simulink model "L400_airframe"  (R2024b)
settings: Solver=FixedStepAuto  StartTime=0  StopTime=20  FixedStep=5/1000  RelTol=1e-3
model workspace (MAT data in the model file):
  Sig : Simulink.Signal (value not decoded)
  Sig1 : Simulink.Signal (value not decoded)
  Sig2 : Simulink.Signal (value not decoded)
  Sig3 : Simulink.Signal (value not decoded)
  Sig4 : Simulink.Signal (value not decoded)
  Sig5 : Simulink.Signal (value not decoded)
  Sig6 : Simulink.Signal (value not decoded)
undefined symbols (not defined in the file or in its folder): convertTo, datetime, db, Earth, F, lambda, Light, MIL, WGS84, WMM2020
libraries: aerolibconvert2 x16, aerolibasang x5, aerolibtransform2 x3, aerolibwind2 x3, aerolibactuator x2, matrix_library x2, shared6dof x1, aerolibatmos2 x1, aerolibgravity2 x1
(part 2 of 4)

== system L400_airframe/actuator/aerodynamic/actuator ==
  BusElementIn1 : Inport  PortName=command  Element=DAL
  BusElementIn : Inport  PortName=command  Element=DAL
  BusElementIn2 : Inport  PortName=command  Element=DER
  BusElementIn3 : Inport  PortName=command  Element=DR
  BusElementIn4 : Inport  PortName=command  Element=DEM
  BusElementIn5 : Inport  PortName=command  Element=DEL
  BusElementIn6 : Inport  PortName=command  Element=DFLO
  BusElementIn7 : Inport  PortName=command  Element=DFLI
  BusElementIn8 : Inport  PortName=command  Element=DFRI
  BusElementIn9 : Inport  PortName=command  Element=DFRO
  Data Type Conversion : DataTypeConversion  SaturateOnIntegerOverflow=off  RndMeth=Floor
  Demux : Demux  Outputs=10
  Mux : Mux  Inputs=10
  Saturation : Saturate  UpperLimit=[30,30,30,30,15,15,17,17,17,23]  LowerLimit=[0,0,0,0,-23,-23,-23,-23,-23,-23]
  Signal Specification4 : SignalSpecification  Unit=deg
  Variant Subsystem : Subsystem  Variant=on
  Bus Element Out : Outport  PortName=surface  Element=DFLO
  Bus Element Out1 : Outport  PortName=surface  Element=DFLI
  Bus Element Out2 : Outport  PortName=surface  Element=DFRI
  Bus Element Out3 : Outport  PortName=surface  Element=DFRO
  Bus Element Out4 : Outport  PortName=surface  Element=DAL
  Bus Element Out5 : Outport  PortName=surface  Element=DAR
  Bus Element Out6 : Outport  PortName=surface  Element=DEL
  Bus Element Out7 : Outport  PortName=surface  Element=DEM
  Bus Element Out8 : Outport  PortName=surface  Element=DER
  Bus Element Out9 : Outport  PortName=surface  Element=DR
  wires:
  Mux/1 -> Data Type Conversion/1
  Saturation/1 -> Signal Specification4/1
  Variant Subsystem/1(Out1) -> Demux/1
  Demux/1 -> Bus Element Out/1
  Demux/2 -> Bus Element Out1/1
  Demux/4 -> Bus Element Out3/1
  Demux/3 -> Bus Element Out2/1
  Signal Specification4/1 -> Variant Subsystem/1(In1)
  BusElementIn6/1 -> Mux/1
  BusElementIn7/1 -> Mux/2
  BusElementIn8/1 -> Mux/3
  BusElementIn9/1 -> Mux/4
  BusElementIn3/1 -> Mux/10
  BusElementIn2/1 -> Mux/9
  BusElementIn5/1 -> Mux/7
  BusElementIn4/1 -> Mux/8
  BusElementIn/1 -> Mux/6
  BusElementIn1/1 -> Mux/5
  Demux/5 -> Bus Element Out4/1
  Demux/6 -> Bus Element Out5/1
  Demux/7 -> Bus Element Out6/1
  Demux/8 -> Bus Element Out7/1
  Demux/9 -> Bus Element Out8/1
  Demux/10 -> Bus Element Out9/1
  Data Type Conversion/1 -> Saturation/1

== system L400_airframe/actuator/aerodynamic/aerodynamics ==
  BusElementIn7 : Inport  PortName=surface
  BusElementIn9 : Inport  Port=2  PortName=state
  BusElementIn4 : Inport  Port=2  PortName=state  Element=aircraft.airdata.qbar
  BusElementIn1 : Inport  Port=2  PortName=state  Element=aircraft.airdata.qbar
  BusElementIn : Inport  Port=2  PortName=state  Element=aircraft.airdata.alpha
  CD : Subsystem
  CL : Subsystem
  CM : Subsystem
  CN : Subsystem
  CR : Subsystem
  CY : Subsystem
  Constant : Constant  Value=db.aerody.COP
  Constant1 : Constant  Value=0
  Direction Cosine Matrix Body to Wind : aerolibtransform2/Direction Cosine Matrix Body to Wind
  Gain : Gain  Gain=db.aerody.Sref
  Gain1 : Gain  Gain=db.aerody.Lref*db.aerody.Sref
  Mux : Mux  Inputs=2
  Mux2 : Mux  Inputs=3
  Mux3 : Mux  Inputs=3
  Product : Product
  Product1 : Product
  Product2 : Product  Multiplication=Matrix(*)
  Transpose : Math  Operator=transpose
  Unary Minus : UnaryMinus
  Unary Minus1 : UnaryMinus
  Bus Element Out : Outport  PortName=aerody  Element=Fxyz
  Bus Element Out1 : Outport  PortName=aerody  Element=Mxyz
  Bus Element Out3 : Outport  PortName=aerody  Element=Pxyz
  wires:
  Constant/1 -> Bus Element Out3/1
  Product1/1 -> Gain1/1
  Product/1 -> Gain/1
  Mux2/1 -> Product1/1  "CR_CM_CN"
  Gain1/1 -> Bus Element Out1/1  "aerody_Mxyz"
  BusElementIn7/1 -> CN/2(surface), CM/2(surface), CR/2(surface), CL/2(surface), CY/2(surface), CD/2(surface)
  [TC] -> CN/1(TC), CM/1(TC), CR/1(TC), CY/1(TC), CL/1(TC), CD/1(TC)
  Direction Cosine Matrix Body to Wind/1 -> Transpose/1
  Transpose/1 -> Product2/1
  Product2/1 -> Product/2
  Mux3/1 -> Product2/2
  Gain/1 -> Bus Element Out/1
  CR/1(CR) -> Mux2/1
  CM/1(CM) -> Mux2/2
  CN/1(CN) -> Mux2/3
  BusElementIn9/1 -> CR/3(state), CN/3(state), CM/3(state), CL/3(state), CY/3(state), CD/3(state)
  CY/1(CY) -> Mux3/2
  CL/1(CL) -> Unary Minus1/1  "CL"
  CD/1(CD) -> Unary Minus/1
  BusElementIn4/1 -> Product1/2
  BusElementIn1/1 -> Product/1
  Unary Minus/1 -> Mux3/1
  Unary Minus1/1 -> Mux3/3
  BusElementIn/1 -> Mux/1
  Constant1/1 -> Mux/2
  Mux/1 -> Direction Cosine Matrix Body to Wind/1

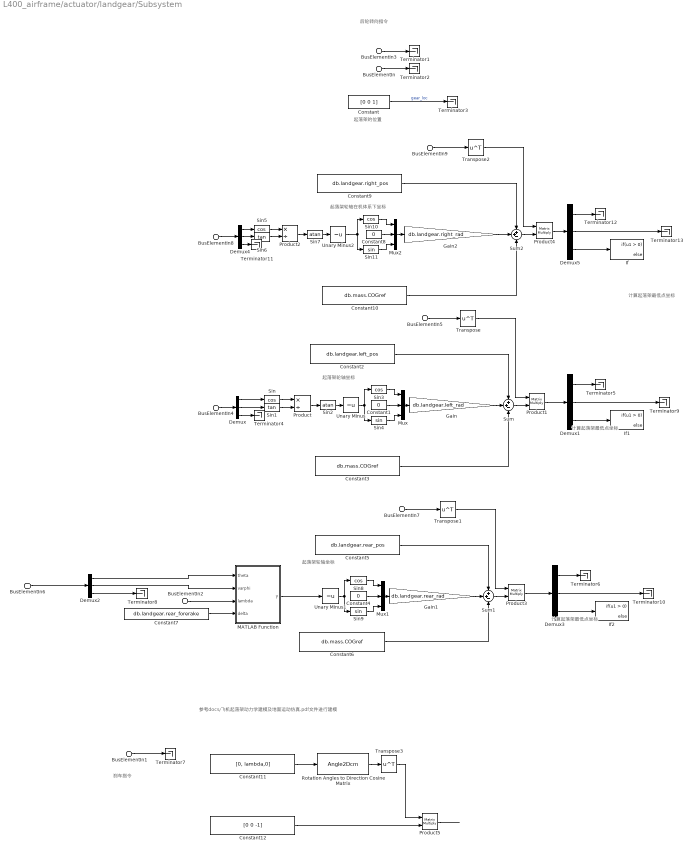
== system L400_airframe/actuator/landgear/Subsystem ==
  note: 起落架轮轴坐标
  note: 计算起落架最低点坐标
  note: 刹车指令
  note: 起落架的位置
  note: 后轮转向指令
  note: 起落架轮轴坐标
  note: 计算起落架最低点坐标
  note: 起落架轮轴在机体系下坐标
  note: 计算起落架最低点坐标
  note: 参考docs/飞机起落架动力学建模及地面运动仿真.pdf文件进行建模
  BusElementIn1 : Inport  PortName=cmd  Element=DB
  BusElementIn2 : Inport  PortName=cmd  Element=DTW
  BusElementIn : Inport  Port=2  PortName=state  Element=aircraft.position.agl
  BusElementIn3 : Inport  Port=2  PortName=state  Element=aircraft.position.alt
  BusElementIn4 : Inport  Port=2  PortName=state  Element=aircraft.attitude.phi_theta_psi
  BusElementIn6 : Inport  Port=2  PortName=state  Element=aircraft.attitude.phi_theta_psi
  BusElementIn8 : Inport  Port=2  PortName=state  Element=aircraft.attitude.phi_theta_psi
  BusElementIn5 : Inport  Port=2  PortName=state  Element=aircraft.attitude.Rbe
  BusElementIn7 : Inport  Port=2  PortName=state  Element=aircraft.attitude.Rbe
  BusElementIn9 : Inport  Port=2  PortName=state  Element=aircraft.attitude.Rbe
  Constant : Constant  Value=[0 0 1]
  Constant1 : Constant  Value=0
  Constant10 : Constant  Value=db.mass.COGref
  Constant11 : Constant  Value=[0, lambda,0]
  Constant12 : Constant  Value=[0 0 -1]
  Constant2 : Constant  Value=db.landgear.left_pos
  Constant3 : Constant  Value=db.mass.COGref
  Constant4 : Constant  Value=0
  Constant5 : Constant  Value=db.landgear.rear_pos
  Constant6 : Constant  Value=db.mass.COGref
  Constant7 : Constant  Value=db.landgear.rear_forerake
  Constant8 : Constant  Value=0
  Constant9 : Constant  Value=db.landgear.right_pos
  Demux : Demux  Outputs=3
  Demux1 : Demux  Outputs=[1,2,3]
  Demux2 : Demux  Outputs=3
  Demux3 : Demux  Outputs=[1,2,3]
  Demux4 : Demux  Outputs=3
  Demux5 : Demux  Outputs=[1,2,3]
  Gain : Gain  Gain=db.landgear.left_rad
  Gain1 : Gain  Gain=db.landgear.rear_rad
  Gain2 : Gain  Gain=db.landgear.right_rad
  If : If
  If1 : If
  If2 : If
  MATLAB Function : MATLAB Function  TreatAsAtomicUnit=on
  Mux : Mux  Inputs=3
  Mux1 : Mux  Inputs=3
  Mux2 : Mux  Inputs=3
  Product : Product  Inputs=*/
  Product{1,3..5} (4 alike) : Product  Multiplication=Matrix(*)
  Product2 : Product  Inputs=*/
  Rotation Angles to Direction Cosine Matrix : Angle2Dcm
      settings: AttributesFormatString=Rotation Order: %<rotationOrder>
  Sin{,3,5,8,10} (5 alike) : Trigonometry  Operator=cos
  Sin1 : Trigonometry  Operator=tan
  Sin11 : Trigonometry
  Sin2 : Trigonometry  Operator=atan
  Sin4 : Trigonometry
  Sin6 : Trigonometry  Operator=tan
  Sin7 : Trigonometry  Operator=atan
  Sin9 : Trigonometry
  Sum : Sum  Inputs=++-
  Sum1 : Sum  Inputs=++-
  Sum2 : Sum  Inputs=++-
  Terminator{1..13} (13 alike) : Terminator
  Transpose{,1..3} (4 alike) : Math  Operator=transpose
  Unary Minus : UnaryMinus
  Unary Minus1 : UnaryMinus
  Unary Minus2 : UnaryMinus
  wires:
  Constant/1 -> Terminator3/1  "gear_loc"
  BusElementIn1/1 -> Terminator7/1
  BusElementIn3/1 -> Terminator1/1
  BusElementIn/1 -> Terminator2/1
  BusElementIn4/1 -> Demux/1
  Demux/2 -> Sin1/1
  Demux/1 -> Sin/1
  Sin/1 -> Product/1
  Sin1/1 -> Product/2
  Product/1 -> Sin2/1
  Demux/3 -> Terminator4/1
  Sin2/1 -> Unary Minus/1
  Constant1/1 -> Mux/2
  Sin3/1 -> Mux/1
  Sin4/1 -> Mux/3
  Mux/1 -> Gain/1
  BusElementIn5/1 -> Transpose/1
  Transpose/1 -> Product1/1
  Sum/1 -> Product1/2
  Unary Minus/1 -> Sin4/1, Sin3/1
  Constant2/1 -> Sum/1
  Gain/1 -> Sum/2
  Constant3/1 -> Sum/3
  Constant6/1 -> Sum1/3
  Gain1/1 -> Sum1/2
  Constant5/1 -> Sum1/1
  Unary Minus1/1 -> Sin8/1, Sin9/1
  Sum1/1 -> Product3/2
  Transpose1/1 -> Product3/1
  BusElementIn7/1 -> Transpose1/1
  Mux1/1 -> Gain1/1
  Sin9/1 -> Mux1/3
  Sin8/1 -> Mux1/1
  Constant4/1 -> Mux1/2
  MATLAB Function/1(y) -> Unary Minus1/1
  Demux2/3 -> Terminator8/1
  Demux2/1 -> MATLAB Function/1(theta)
  Demux2/2 -> MATLAB Function/2(varphi)
  BusElementIn6/1 -> Demux2/1
  BusElementIn2/1 -> MATLAB Function/3(lambda)
  Constant7/1 -> MATLAB Function/4(delta)
  Demux5/2 -> Terminator13/1
  Demux5/1 -> Terminator12/1
  Product4/1 -> Demux5/1
  Constant10/1 -> Sum2/3
  Gain2/1 -> Sum2/2
  Constant9/1 -> Sum2/1
  Unary Minus2/1 -> Sin10/1, Sin11/1
  Sum2/1 -> Product4/2
  Transpose2/1 -> Product4/1
  BusElementIn9/1 -> Transpose2/1
  Mux2/1 -> Gain2/1
  Sin11/1 -> Mux2/3
  Sin10/1 -> Mux2/1
  Constant8/1 -> Mux2/2
  Sin7/1 -> Unary Minus2/1
  Demux4/3 -> Terminator11/1
  Product2/1 -> Sin7/1
  Sin6/1 -> Product2/2
  Sin5/1 -> Product2/1
  Demux4/1 -> Sin5/1
  Demux4/2 -> Sin6/1
  BusElementIn8/1 -> Demux4/1
  Demux5/3 -> If/1
  Demux1/3 -> If1/1
  Product1/1 -> Demux1/1
  Demux1/1 -> Terminator5/1
  Demux1/2 -> Terminator9/1
  Demux3/2 -> Terminator10/1
  Demux3/1 -> Terminator6/1
  Demux3/3 -> If2/1
  Product3/1 -> Demux3/1
  Constant11/1 -> Rotation Angles to Direction Cosine Matrix/1
  Rotation Angles to Direction Cosine Matrix/1 -> Transpose3/1
  Constant12/1 -> Product5/2
  Transpose3/1 -> Product5/1
  Product5/1 -> ?

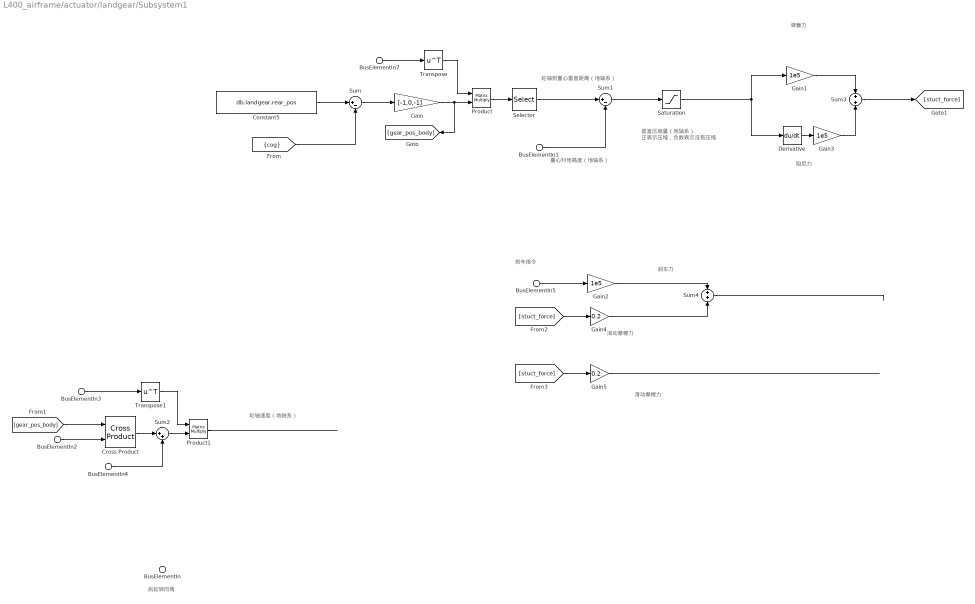
== system L400_airframe/actuator/landgear/Subsystem1 ==
  note: 滚动摩檫力
  note: 后轮转向角
  note: 刹车力
  note: 滑动摩檫力
  note: 轮轴速度（地轴系）
  note: 垂直压缩量（地轴系）
      | 正表示压缩，负数表示没有压缩
  note: 轮轴到重心垂直距离（地轴系）
  note: 重心对地高度（地轴系）
  note: 刹车指令
  note: 弹簧力
  note: 阻尼力
  BusElementIn5 : Inport  PortName=cmd  Element=DB
  BusElementIn : Inport  PortName=cmd  Element=DTW
  BusElementIn7 : Inport  Port=2  PortName=state  Element=aircraft.attitude.Rbe
  BusElementIn3 : Inport  Port=2  PortName=state  Element=aircraft.attitude.Rbe
  BusElementIn2 : Inport  Port=2  PortName=state  Element=aircraft.attitude.p_q_r
  BusElementIn1 : Inport  Port=2  PortName=state  Element=aircraft.position.agl
  BusElementIn4 : Inport  Port=2  PortName=state  Element=aircraft.position.vx_vy_vz
  Constant5 : Constant  Value=db.landgear.rear_pos
  Cross Product : matrix_library/Cross Product
  Derivative : Derivative
  Gain : Gain  Gain=[-1,0,-1]
  Gain1 : Gain  Gain=1e5
  Gain2 : Gain  Gain=1e5
  Gain3 : Gain  Gain=1e5
  Gain4 : Gain  Gain=0.2
  Gain5 : Gain  Gain=0.2
  Product : Product  Multiplication=Matrix(*)
  Product1 : Product  Multiplication=Matrix(*)
  Saturation : Saturate  UpperLimit=inf  LowerLimit=0
  Selector : Selector  InputPortWidth=3  IndexOptions=Index vector (dialog)  Indices=3  OutputSizes=1
  Sum : Sum  Inputs=|+-
  Sum1 : Sum  Inputs=|+-
  Sum2 : Sum  Inputs=|++
  Sum3 : Sum  Inputs=2
  Sum4 : Sum  Inputs=2
  Transpose : Math  Operator=transpose
  Transpose1 : Math  Operator=transpose
  wires:
  [cog] -> Sum/2
  Constant5/1 -> Sum/1
  Sum/1 -> Gain/1
  Gain/1 -> [gear_pos_body], Product/2
  BusElementIn7/1 -> Transpose/1
  Transpose/1 -> Product/1
  Product/1 -> Selector/1
  Selector/1 -> Sum1/1
  BusElementIn1/1 -> Sum1/2
  Sum1/1 -> Saturation/1
  Saturation/1 -> Derivative/1, Gain1/1
  [gear_pos_body] -> Cross Product/1
  BusElementIn2/1 -> Cross Product/2
  Transpose1/1 -> Product1/1
  BusElementIn3/1 -> Transpose1/1
  Product1/1 -> ?
  Cross Product/1 -> Sum2/1
  BusElementIn4/1 -> Sum2/2
  Sum2/1 -> Product1/2
  BusElementIn5/1 -> Gain2/1
  Derivative/1 -> Gain3/1
  Sum3/1 -> [stuct_force]
  Gain4/1 -> Sum4/2
  [stuct_force] -> Gain4/1
  Gain2/1 -> Sum4/1
  Sum4/1 -> ?
  [stuct_force] -> Gain5/1
  Gain5/1 -> ?
  Gain3/1 -> Sum3/2
  Gain1/1 -> Sum3/1

== system L400_airframe/force/Subsystem1/For Each Subsystem ==
  Fxyz : Inport  Partition=on  PartitionDimension=2  PartitionWidth=1  PartitionOffset=0
  Mxyz : Inport  Port=2  Partition=on  PartitionDimension=2  PartitionWidth=1  PartitionOffset=0
  Pxyz : Inport  Port=3  Partition=on  PartitionDimension=2  PartitionWidth=1  PartitionOffset=0
  COG : Inport  Port=4
  Cross Product : matrix_library/Cross Product
  For Each : ForEach  DisableCoverage=on
  Gain : Gain  Gain=[-1 1 -1]
  Sum : Sum  Inputs=|+-
  Sum1 : Sum  Inputs=|++
  M : Outport  ConcatenationDimension=2
  wires:
  Mxyz/1 -> Sum1/2
  Sum/1 -> Gain/1
  Fxyz/1 -> Cross Product/2
  Sum1/1 -> M/1
  Cross Product/1 -> Sum1/1
  Pxyz/1 -> Sum/1
  COG/1 -> Sum/2
  Gain/1 -> Cross Product/1

== system L400_airframe/sensor/gps/posix time ==
  Clock : Clock
  Constant : Constant  Value=convertTo(datetime('now','TimeZone','UTC'),'posixtime')
  Gain : Gain  Gain=1e6  OutDataTypeStr=uint64
  Sum : Sum  Inputs=|++
  utc : Outport  Unit=µs
  wires:
  Clock/1 -> Sum/1
  Sum/1 -> Gain/1
  Constant/1 -> Sum/2
  Gain/1 -> utc/1

== system L400_airframe/state/Variant Subsystem/Subsystem ==
  h(m) : Inport
  μ(deg) : Inport  Port=2
  l(deg) : Inport  Port=3
  Constant : Constant  Value=[1 0 0]
  Constant1 : Constant  Value=0
  Terminator : Terminator
  Terminator1 : Terminator
  Terminator2 : Terminator
  XYZ(nT) : Outport
  H(nT) : Outport  Port=2
  D(deg) : Outport  Port=3
  I(deg) : Outport  Port=4
  F(nT) : Outport  Port=5
  wires:
  h(m)/1 -> Terminator/1
  l(deg)/1 -> Terminator2/1
  μ(deg)/1 -> Terminator1/1
  Constant/1 -> XYZ(nT)/1
  Constant1/1 -> F(nT)/1, I(deg)/1, H(nT)/1, D(deg)/1

== system L400_airframe/state/Variant Subsystem/Subsystem1 ==
  h(m) : Inport
  μ(deg) : Inport  Port=2
  l(deg) : Inport  Port=3
  World Magnetic Model : aerolibgravity2/World Magnetic Model  model=WMM2020 (2020-2025)  customFile='WMM2020.COF'  units=Metric (MKS)  time_in=off  month=January  day=1  year=2020  action=Error  h_out=on  dec_out=on  inc_out=on  ti_out=on
  XYZ(nT) : Outport
  H(nT) : Outport  Port=2
  D(deg) : Outport  Port=3
  I(deg) : Outport  Port=4
  F(nT) : Outport  Port=5
  wires:
  h(m)/1 -> World Magnetic Model/1
  World Magnetic Model/1 -> XYZ(nT)/1
  World Magnetic Model/2 -> H(nT)/1
  World Magnetic Model/3 -> D(deg)/1
  World Magnetic Model/4 -> I(deg)/1
  World Magnetic Model/5 -> F(nT)/1
  l(deg)/1 -> World Magnetic Model/3
  μ(deg)/1 -> World Magnetic Model/2

== system L400_airframe/actuator/aerodynamic/actuator/Variant Subsystem ==
  note: 1) Add Subsystem or Model blocks as valid variant choices.
      | 2) You cannot connect blocks at this level. At simulation, connectivity is automatically
      | determined, based on the active variant and port name matching.
  In1 : Inport
  Subsystem : Subsystem  VariantControl=true
  Subsystem1 : Subsystem  VariantControl=false
  Out1 : Outport

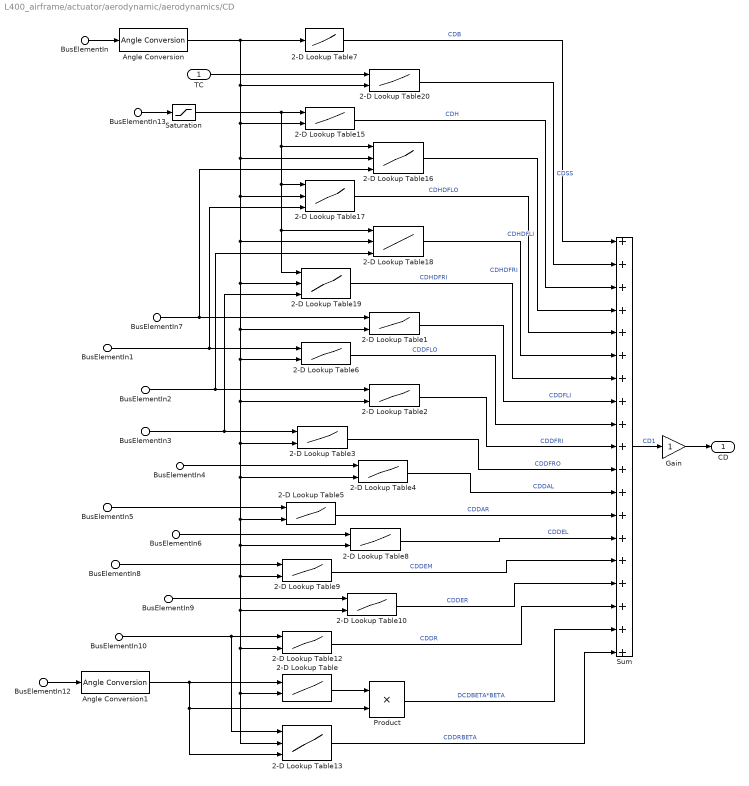
== system L400_airframe/actuator/aerodynamic/aerodynamics/CD ==
  TC : Inport
  BusElementIn7 : Inport  Port=2  PortName=surface  Element=DFLI
  BusElementIn1 : Inport  Port=2  PortName=surface  Element=DFLO
  BusElementIn2 : Inport  Port=2  PortName=surface  Element=DFRI
  BusElementIn3 : Inport  Port=2  PortName=surface  Element=DFRO
  BusElementIn4 : Inport  Port=2  PortName=surface  Element=DAL
  BusElementIn5 : Inport  Port=2  PortName=surface  Element=DAR
  BusElementIn6 : Inport  Port=2  PortName=surface  Element=DEL
  BusElementIn8 : Inport  Port=2  PortName=surface  Element=DEM
  BusElementIn9 : Inport  Port=2  PortName=surface  Element=DER
  BusElementIn10 : Inport  Port=2  PortName=surface  Element=DR
  BusElementIn : Inport  Port=3  PortName=state  Element=aircraft.airdata.alpha
  BusElementIn12 : Inport  Port=3  PortName=state  Element=aircraft.airdata.beta
  BusElementIn13 : Inport  Port=3  PortName=state  Element=aircraft.position.agl
  2-D Lookup Table : Lookup_n-D  LookupTableObject=''  BreakpointsForDimension1=db.aerody.VBETA  BreakpointsForDimension2=db.aerody.VALPHA  BreakpointsForDimension1FirstPoint=10  BreakpointsForDimension2FirstPoint=10  BreakpointsForDimension1Spacing=12  BreakpointsForDimension2Spacing=12  IndexSearchMethod=Linear search  BeginIndexSearchUsingPreviousIndexResult=on  Table=db.aerody.DCDBETA  ExtrapMethod=Clip  DiagnosticForOutOfRangeInput=Warning  InternalRulePriority=Speed  RndMeth=Simplest
      settings: InputPortMap=u0,u1
  2-D Lookup Table1 : Lookup_n-D  LookupTableObject=''  BreakpointsForDimension1=db.aerody.VDF  BreakpointsForDimension2=db.aerody.VALPHA  BreakpointsForDimension1FirstPoint=10  BreakpointsForDimension2FirstPoint=10  BreakpointsForDimension1Spacing=12  BreakpointsForDimension2Spacing=12  IndexSearchMethod=Linear search  BeginIndexSearchUsingPreviousIndexResult=on  Table=db.aerody.CDDFLI  ExtrapMethod=Clip  DiagnosticForOutOfRangeInput=Warning  InternalRulePriority=Speed  RndMeth=Simplest
      settings: InputPortMap=u0,u1
  2-D Lookup Table10 : Lookup_n-D  LookupTableObject=''  BreakpointsForDimension1=db.aerody.VDE  BreakpointsForDimension2=db.aerody.VALPHA  BreakpointsForDimension1FirstPoint=10  BreakpointsForDimension2FirstPoint=10  BreakpointsForDimension1Spacing=12  BreakpointsForDimension2Spacing=12  IndexSearchMethod=Linear search  BeginIndexSearchUsingPreviousIndexResult=on  Table=db.aerody.CDDER  ExtrapMethod=Clip  DiagnosticForOutOfRangeInput=Warning  InternalRulePriority=Speed  RndMeth=Simplest
      settings: InputPortMap=u0,u1
  2-D Lookup Table12 : Lookup_n-D  LookupTableObject=''  BreakpointsForDimension1=db.aerody.VDR  BreakpointsForDimension2=db.aerody.VALPHA  BreakpointsForDimension1FirstPoint=10  BreakpointsForDimension2FirstPoint=10  BreakpointsForDimension1Spacing=12  BreakpointsForDimension2Spacing=12  IndexSearchMethod=Linear search  BeginIndexSearchUsingPreviousIndexResult=on  Table=db.aerody.CDDR  ExtrapMethod=Clip  DiagnosticForOutOfRangeInput=Warning  InternalRulePriority=Speed  RndMeth=Simplest
      settings: InputPortMap=u0,u1
  2-D Lookup Table13 : Lookup_n-D  NumberOfTableDimensions=3  LookupTableObject=''  BreakpointsForDimension1=db.aerody.VDR  BreakpointsForDimension2=db.aerody.VALPHA  BreakpointsForDimension3=db.aerody.VBETA  BreakpointsForDimension1FirstPoint=10  BreakpointsForDimension2FirstPoint=10  BreakpointsForDimension1Spacing=12  BreakpointsForDimension2Spacing=12  IndexSearchMethod=Linear search  BeginIndexSearchUsingPreviousIndexResult=on  Table=db.aerody.CDDRBETA  ExtrapMethod=Clip  DiagnosticForOutOfRangeInput=Warning  InternalRulePriority=Speed  RndMeth=Simplest
      settings: InputPortMap=u0,u1,u2
  2-D Lookup Table15 : Lookup_n-D  LookupTableObject=''  BreakpointsForDimension1=db.aerody.VH  BreakpointsForDimension2=db.aerody.VALPHA  BreakpointsForDimension1FirstPoint=10  BreakpointsForDimension2FirstPoint=10  BreakpointsForDimension1Spacing=12  BreakpointsForDimension2Spacing=12  IndexSearchMethod=Linear search  BeginIndexSearchUsingPreviousIndexResult=on  Table=db.aerody.CDH  ExtrapMethod=Clip  DiagnosticForOutOfRangeInput=Warning  InternalRulePriority=Speed  RndMeth=Simplest
      settings: InputPortMap=u0,u1
  2-D Lookup Table16 : Lookup_n-D  NumberOfTableDimensions=3  LookupTableObject=''  BreakpointsForDimension1=db.aerody.VH  BreakpointsForDimension2=db.aerody.VALPHA  BreakpointsForDimension3=db.aerody.VDF  BreakpointsForDimension1FirstPoint=10  BreakpointsForDimension2FirstPoint=10  BreakpointsForDimension1Spacing=12  BreakpointsForDimension2Spacing=12  IndexSearchMethod=Linear search  BeginIndexSearchUsingPreviousIndexResult=on  Table=db.aerody.CDHDFLI  ExtrapMethod=Clip  DiagnosticForOutOfRangeInput=Warning  InternalRulePriority=Speed  RndMeth=Simplest
      settings: InputPortMap=u0,u1,u2
  2-D Lookup Table17 : Lookup_n-D  NumberOfTableDimensions=3  LookupTableObject=''  BreakpointsForDimension1=db.aerody.VH  BreakpointsForDimension2=db.aerody.VALPHA  BreakpointsForDimension3=db.aerody.VDF  BreakpointsForDimension1FirstPoint=10  BreakpointsForDimension2FirstPoint=10  BreakpointsForDimension1Spacing=12  BreakpointsForDimension2Spacing=12  IndexSearchMethod=Linear search  BeginIndexSearchUsingPreviousIndexResult=on  Table=db.aerody.CDHDFLO  ExtrapMethod=Clip  DiagnosticForOutOfRangeInput=Warning  InternalRulePriority=Speed  RndMeth=Simplest
      settings: InputPortMap=u0,u1,u2
  2-D Lookup Table18 : Lookup_n-D  NumberOfTableDimensions=3  LookupTableObject=''  BreakpointsForDimension1=db.aerody.VH  BreakpointsForDimension2=db.aerody.VALPHA  BreakpointsForDimension3=db.aerody.VDF  BreakpointsForDimension1FirstPoint=10  BreakpointsForDimension2FirstPoint=10  BreakpointsForDimension1Spacing=12  BreakpointsForDimension2Spacing=12  IndexSearchMethod=Linear search  BeginIndexSearchUsingPreviousIndexResult=on  Table=db.aerody.CDHDFRI  ExtrapMethod=Clip  DiagnosticForOutOfRangeInput=Warning  InternalRulePriority=Speed  RndMeth=Simplest
      settings: InputPortMap=u0,u1,u2
  2-D Lookup Table19 : Lookup_n-D  NumberOfTableDimensions=3  LookupTableObject=''  BreakpointsForDimension1=db.aerody.VH  BreakpointsForDimension2=db.aerody.VALPHA  BreakpointsForDimension3=db.aerody.VDF  BreakpointsForDimension1FirstPoint=10  BreakpointsForDimension2FirstPoint=10  BreakpointsForDimension1Spacing=12  BreakpointsForDimension2Spacing=12  IndexSearchMethod=Linear search  BeginIndexSearchUsingPreviousIndexResult=on  Table=db.aerody.CDHDFRO  ExtrapMethod=Clip  DiagnosticForOutOfRangeInput=Warning  InternalRulePriority=Speed  RndMeth=Simplest
      settings: InputPortMap=u0,u1,u2
  2-D Lookup Table2 : Lookup_n-D  LookupTableObject=''  BreakpointsForDimension1=db.aerody.VDF  BreakpointsForDimension2=db.aerody.VALPHA  BreakpointsForDimension1FirstPoint=10  BreakpointsForDimension2FirstPoint=10  BreakpointsForDimension1Spacing=12  BreakpointsForDimension2Spacing=12  IndexSearchMethod=Linear search  BeginIndexSearchUsingPreviousIndexResult=on  Table=db.aerody.CDDFRI  ExtrapMethod=Clip  DiagnosticForOutOfRangeInput=Warning  InternalRulePriority=Speed  RndMeth=Simplest
      settings: InputPortMap=u0,u1
  2-D Lookup Table20 : Lookup_n-D  LookupTableObject=''  BreakpointsForDimension1=db.aerody.VTC  BreakpointsForDimension2=db.aerody.VALPHA  BreakpointsForDimension1FirstPoint=10  BreakpointsForDimension2FirstPoint=10  BreakpointsForDimension1Spacing=12  BreakpointsForDimension2Spacing=12  IndexSearchMethod=Linear search  BeginIndexSearchUsingPreviousIndexResult=on  Table=db.aerody.CDSS  ExtrapMethod=Clip  DiagnosticForOutOfRangeInput=Warning  InternalRulePriority=Speed  RndMeth=Simplest
      settings: InputPortMap=u0,u1
  2-D Lookup Table3 : Lookup_n-D  LookupTableObject=''  BreakpointsForDimension1=db.aerody.VDF  BreakpointsForDimension2=db.aerody.VALPHA  BreakpointsForDimension1FirstPoint=10  BreakpointsForDimension2FirstPoint=10  BreakpointsForDimension1Spacing=12  BreakpointsForDimension2Spacing=12  IndexSearchMethod=Linear search  BeginIndexSearchUsingPreviousIndexResult=on  Table=db.aerody.CDDFRO  ExtrapMethod=Clip  DiagnosticForOutOfRangeInput=Warning  InternalRulePriority=Speed  RndMeth=Simplest
      settings: InputPortMap=u0,u1
  2-D Lookup Table4 : Lookup_n-D  LookupTableObject=''  BreakpointsForDimension1=db.aerody.VDA  BreakpointsForDimension2=db.aerody.VALPHA  BreakpointsForDimension1FirstPoint=10  BreakpointsForDimension2FirstPoint=10  BreakpointsForDimension1Spacing=12  BreakpointsForDimension2Spacing=12  IndexSearchMethod=Linear search  BeginIndexSearchUsingPreviousIndexResult=on  Table=db.aerody.CDDAL  ExtrapMethod=Clip  DiagnosticForOutOfRangeInput=Warning  InternalRulePriority=Speed  RndMeth=Simplest
      settings: InputPortMap=u0,u1
  2-D Lookup Table5 : Lookup_n-D  LookupTableObject=''  BreakpointsForDimension1=db.aerody.VDA  BreakpointsForDimension2=db.aerody.VALPHA  BreakpointsForDimension1FirstPoint=10  BreakpointsForDimension2FirstPoint=10  BreakpointsForDimension1Spacing=12  BreakpointsForDimension2Spacing=12  IndexSearchMethod=Linear search  BeginIndexSearchUsingPreviousIndexResult=on  Table=db.aerody.CDDAR  ExtrapMethod=Clip  DiagnosticForOutOfRangeInput=Warning  InternalRulePriority=Speed  RndMeth=Simplest
      settings: InputPortMap=u0,u1
  2-D Lookup Table6 : Lookup_n-D  LookupTableObject=''  BreakpointsForDimension1=db.aerody.VDF  BreakpointsForDimension2=db.aerody.VALPHA  BreakpointsForDimension1FirstPoint=10  BreakpointsForDimension2FirstPoint=10  BreakpointsForDimension1Spacing=12  BreakpointsForDimension2Spacing=12  IndexSearchMethod=Linear search  BeginIndexSearchUsingPreviousIndexResult=on  Table=db.aerody.CDDFLO  ExtrapMethod=Clip  DiagnosticForOutOfRangeInput=Warning  InternalRulePriority=Speed  RndMeth=Simplest
      settings: InputPortMap=u0,u1
  2-D Lookup Table7 : Lookup_n-D  NumberOfTableDimensions=1  LookupTableObject=''  BreakpointsForDimension1=db.aerody.VALPHA  BreakpointsForDimension2=aerody.basic.cx.beta  BreakpointsForDimension1FirstPoint=10  BreakpointsForDimension2FirstPoint=10  BreakpointsForDimension1Spacing=12  BreakpointsForDimension2Spacing=12  IndexSearchMethod=Linear search  BeginIndexSearchUsingPreviousIndexResult=on  Table=db.aerody.CDB  ExtrapMethod=Clip  DiagnosticForOutOfRangeInput=Warning  InternalRulePriority=Speed  RndMeth=Simplest
  2-D Lookup Table8 : Lookup_n-D  LookupTableObject=''  BreakpointsForDimension1=db.aerody.VDE  BreakpointsForDimension2=db.aerody.VALPHA  BreakpointsForDimension1FirstPoint=10  BreakpointsForDimension2FirstPoint=10  BreakpointsForDimension1Spacing=12  BreakpointsForDimension2Spacing=12  IndexSearchMethod=Linear search  BeginIndexSearchUsingPreviousIndexResult=on  Table=db.aerody.CDDEL  ExtrapMethod=Clip  DiagnosticForOutOfRangeInput=Warning  InternalRulePriority=Speed  RndMeth=Simplest
      settings: InputPortMap=u0,u1
  2-D Lookup Table9 : Lookup_n-D  LookupTableObject=''  BreakpointsForDimension1=db.aerody.VDE  BreakpointsForDimension2=db.aerody.VALPHA  BreakpointsForDimension1FirstPoint=10  BreakpointsForDimension2FirstPoint=10  BreakpointsForDimension1Spacing=12  BreakpointsForDimension2Spacing=12  IndexSearchMethod=Linear search  BeginIndexSearchUsingPreviousIndexResult=on  Table=db.aerody.CDDEM  ExtrapMethod=Clip  DiagnosticForOutOfRangeInput=Warning  InternalRulePriority=Speed  RndMeth=Simplest
      settings: InputPortMap=u0,u1
  Angle Conversion : aerolibconvert2/Angle Conversion  IU=rad  OU=deg
  Angle Conversion1 : aerolibconvert2/Angle Conversion  IU=rad  OU=deg
  Gain : Gain
  Product : Product
  Saturation : Saturate  UpperLimit=5.8  LowerLimit=0
  Sum : Sum  Inputs=19
  CD : Outport
  wires:
  BusElementIn/1 -> Angle Conversion/1
  TC/1 -> 2-D Lookup Table20/1
  BusElementIn13/1 -> Saturation/1
  2-D Lookup Table/1 -> Product/1
  BusElementIn12/1 -> Angle Conversion1/1
  BusElementIn10/1 -> 2-D Lookup Table13/1, 2-D Lookup Table12/1
  BusElementIn9/1 -> 2-D Lookup Table10/1
  BusElementIn8/1 -> 2-D Lookup Table9/1
  BusElementIn6/1 -> 2-D Lookup Table8/1
  BusElementIn5/1 -> 2-D Lookup Table5/1
  BusElementIn4/1 -> 2-D Lookup Table4/1
  BusElementIn3/1 -> 2-D Lookup Table19/3, 2-D Lookup Table3/1
  BusElementIn2/1 -> 2-D Lookup Table18/3, 2-D Lookup Table2/1
  BusElementIn1/1 -> 2-D Lookup Table17/3, 2-D Lookup Table6/1
  BusElementIn7/1 -> 2-D Lookup Table16/3, 2-D Lookup Table1/1
  Sum/1 -> Gain/1  "CD1"
  2-D Lookup Table4/1 -> Sum/12  "CDDAL"
  2-D Lookup Table8/1 -> Sum/14  "CDDEL"
  2-D Lookup Table2/1 -> Sum/10  "CDDFRI"
  2-D Lookup Table1/1 -> Sum/8  "CDDFLI"
  2-D Lookup Table10/1 -> Sum/16  "CDDER"
  2-D Lookup Table5/1 -> Sum/13  "CDDAR"
  2-D Lookup Table3/1 -> Sum/11  "CDDFRO"
  2-D Lookup Table18/1 -> Sum/6  "CDHDFRI"
  2-D Lookup Table9/1 -> Sum/15  "CDDEM"
  2-D Lookup Table6/1 -> Sum/9  "CDDFLO"
  2-D Lookup Table16/1 -> Sum/4  "CDHDFLI"
  Product/1 -> Sum/18  "DCDBETA*BETA"
  2-D Lookup Table12/1 -> Sum/17  "CDDR"
  2-D Lookup Table19/1 -> Sum/7  "CDHDFRI"
  2-D Lookup Table20/1 -> Sum/2  "CDSS"
  2-D Lookup Table17/1 -> Sum/5  "CDHDFLO"
  2-D Lookup Table15/1 -> Sum/3  "CDH"
  2-D Lookup Table13/1 -> Sum/19  "CDDRBETA"
  2-D Lookup Table7/1 -> Sum/1  "CDB"
  Gain/1 -> CD/1
  Angle Conversion/1 -> 2-D Lookup Table7/1, 2-D Lookup Table20/2, 2-D Lookup Table15/2, 2-D Lookup Table16/2, 2-D Lookup Table17/2, 2-D Lookup Table18/2, 2-D Lookup Table19/2, 2-D Lookup Table1/2, 2-D Lookup Table6/2, 2-D Lookup Table2/2, 2-D Lookup Table/2, 2-D Lookup Table13/2, 2-D Lookup Table12/2, 2-D Lookup Table10/2, 2-D Lookup Table9/2, 2-D Lookup Table8/2, 2-D Lookup Table5/2, 2-D Lookup Table4/2, 2-D Lookup Table3/2
  Saturation/1 -> 2-D Lookup Table15/1, 2-D Lookup Table16/1, 2-D Lookup Table17/1, 2-D Lookup Table18/1, 2-D Lookup Table19/1
  Angle Conversion1/1 -> 2-D Lookup Table13/3, Product/2, 2-D Lookup Table/1

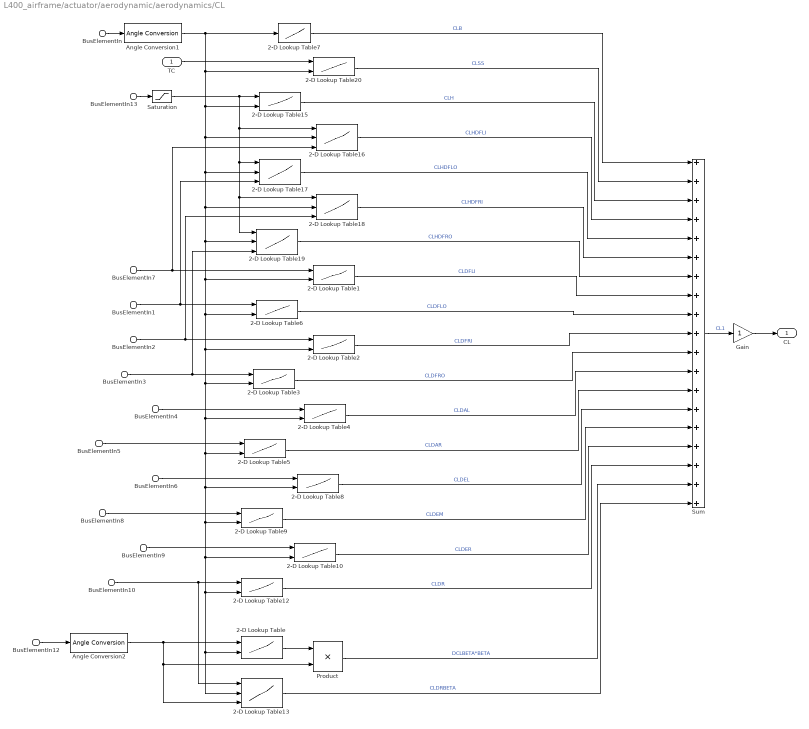
== system L400_airframe/actuator/aerodynamic/aerodynamics/CL ==
  TC : Inport
  BusElementIn7 : Inport  Port=2  PortName=surface  Element=DFLI
  BusElementIn1 : Inport  Port=2  PortName=surface  Element=DFLO
  BusElementIn2 : Inport  Port=2  PortName=surface  Element=DFRI
  BusElementIn3 : Inport  Port=2  PortName=surface  Element=DFRO
  BusElementIn4 : Inport  Port=2  PortName=surface  Element=DAL
  BusElementIn5 : Inport  Port=2  PortName=surface  Element=DAR
  BusElementIn6 : Inport  Port=2  PortName=surface  Element=DEL
  BusElementIn8 : Inport  Port=2  PortName=surface  Element=DEM
  BusElementIn9 : Inport  Port=2  PortName=surface  Element=DER
  BusElementIn10 : Inport  Port=2  PortName=surface  Element=DR
  BusElementIn : Inport  Port=3  PortName=state  Element=aircraft.airdata.alpha
  BusElementIn12 : Inport  Port=3  PortName=state  Element=aircraft.airdata.beta
  BusElementIn13 : Inport  Port=3  PortName=state  Element=aircraft.position.agl
  2-D Lookup Table : Lookup_n-D  LookupTableObject=''  BreakpointsForDimension1=db.aerody.VBETA  BreakpointsForDimension2=db.aerody.VALPHA  BreakpointsForDimension1FirstPoint=10  BreakpointsForDimension2FirstPoint=10  BreakpointsForDimension1Spacing=12  BreakpointsForDimension2Spacing=12  IndexSearchMethod=Linear search  BeginIndexSearchUsingPreviousIndexResult=on  Table=db.aerody.DCLBETA  ExtrapMethod=Clip  DiagnosticForOutOfRangeInput=Warning  InternalRulePriority=Speed  RndMeth=Simplest
      settings: InputPortMap=u0,u1
  2-D Lookup Table1 : Lookup_n-D  LookupTableObject=''  BreakpointsForDimension1=db.aerody.VDF  BreakpointsForDimension2=db.aerody.VALPHA  BreakpointsForDimension1FirstPoint=10  BreakpointsForDimension2FirstPoint=10  BreakpointsForDimension1Spacing=12  BreakpointsForDimension2Spacing=12  IndexSearchMethod=Linear search  BeginIndexSearchUsingPreviousIndexResult=on  Table=db.aerody.CLDFLI  ExtrapMethod=Clip  DiagnosticForOutOfRangeInput=Warning  InternalRulePriority=Speed  RndMeth=Simplest
      settings: InputPortMap=u0,u1
  2-D Lookup Table10 : Lookup_n-D  LookupTableObject=''  BreakpointsForDimension1=db.aerody.VDE  BreakpointsForDimension2=db.aerody.VALPHA  BreakpointsForDimension1FirstPoint=10  BreakpointsForDimension2FirstPoint=10  BreakpointsForDimension1Spacing=12  BreakpointsForDimension2Spacing=12  IndexSearchMethod=Linear search  BeginIndexSearchUsingPreviousIndexResult=on  Table=db.aerody.CLDER  ExtrapMethod=Clip  DiagnosticForOutOfRangeInput=Warning  InternalRulePriority=Speed  RndMeth=Simplest
      settings: InputPortMap=u0,u1
  2-D Lookup Table12 : Lookup_n-D  LookupTableObject=''  BreakpointsForDimension1=db.aerody.VDR  BreakpointsForDimension2=db.aerody.VALPHA  BreakpointsForDimension1FirstPoint=10  BreakpointsForDimension2FirstPoint=10  BreakpointsForDimension1Spacing=12  BreakpointsForDimension2Spacing=12  IndexSearchMethod=Linear search  BeginIndexSearchUsingPreviousIndexResult=on  Table=db.aerody.CLDR  ExtrapMethod=Clip  DiagnosticForOutOfRangeInput=Warning  InternalRulePriority=Speed  RndMeth=Simplest
      settings: InputPortMap=u0,u1
  2-D Lookup Table13 : Lookup_n-D  NumberOfTableDimensions=3  LookupTableObject=''  BreakpointsForDimension1=db.aerody.VDR  BreakpointsForDimension2=db.aerody.VALPHA  BreakpointsForDimension3=db.aerody.VBETA  BreakpointsForDimension1FirstPoint=10  BreakpointsForDimension2FirstPoint=10  BreakpointsForDimension1Spacing=12  BreakpointsForDimension2Spacing=12  IndexSearchMethod=Linear search  BeginIndexSearchUsingPreviousIndexResult=on  Table=db.aerody.CLDRBETA  ExtrapMethod=Clip  DiagnosticForOutOfRangeInput=Warning  InternalRulePriority=Speed  RndMeth=Simplest
      settings: InputPortMap=u0,u1,u2
  2-D Lookup Table15 : Lookup_n-D  LookupTableObject=''  BreakpointsForDimension1=db.aerody.VH  BreakpointsForDimension2=db.aerody.VALPHA  BreakpointsForDimension1FirstPoint=10  BreakpointsForDimension2FirstPoint=10  BreakpointsForDimension1Spacing=12  BreakpointsForDimension2Spacing=12  IndexSearchMethod=Linear search  BeginIndexSearchUsingPreviousIndexResult=on  Table=db.aerody.CLH  ExtrapMethod=Clip  DiagnosticForOutOfRangeInput=Warning  InternalRulePriority=Speed  RndMeth=Simplest
      settings: InputPortMap=u0,u1
  2-D Lookup Table16 : Lookup_n-D  NumberOfTableDimensions=3  LookupTableObject=''  BreakpointsForDimension1=db.aerody.VH  BreakpointsForDimension2=db.aerody.VALPHA  BreakpointsForDimension3=db.aerody.VDF  BreakpointsForDimension1FirstPoint=10  BreakpointsForDimension2FirstPoint=10  BreakpointsForDimension1Spacing=12  BreakpointsForDimension2Spacing=12  IndexSearchMethod=Linear search  BeginIndexSearchUsingPreviousIndexResult=on  Table=db.aerody.CLHDFLI  ExtrapMethod=Clip  DiagnosticForOutOfRangeInput=Warning  InternalRulePriority=Speed  RndMeth=Simplest
      settings: InputPortMap=u0,u1,u2
  2-D Lookup Table17 : Lookup_n-D  NumberOfTableDimensions=3  LookupTableObject=''  BreakpointsForDimension1=db.aerody.VH  BreakpointsForDimension2=db.aerody.VALPHA  BreakpointsForDimension3=db.aerody.VDF  BreakpointsForDimension1FirstPoint=10  BreakpointsForDimension2FirstPoint=10  BreakpointsForDimension1Spacing=12  BreakpointsForDimension2Spacing=12  IndexSearchMethod=Linear search  BeginIndexSearchUsingPreviousIndexResult=on  Table=db.aerody.CLHDFLO  ExtrapMethod=Clip  DiagnosticForOutOfRangeInput=Warning  InternalRulePriority=Speed  RndMeth=Simplest
      settings: InputPortMap=u0,u1,u2
  2-D Lookup Table18 : Lookup_n-D  NumberOfTableDimensions=3  LookupTableObject=''  BreakpointsForDimension1=db.aerody.VH  BreakpointsForDimension2=db.aerody.VALPHA  BreakpointsForDimension3=db.aerody.VDF  BreakpointsForDimension1FirstPoint=10  BreakpointsForDimension2FirstPoint=10  BreakpointsForDimension1Spacing=12  BreakpointsForDimension2Spacing=12  IndexSearchMethod=Linear search  BeginIndexSearchUsingPreviousIndexResult=on  Table=db.aerody.CLHDFRI  ExtrapMethod=Clip  DiagnosticForOutOfRangeInput=Warning  InternalRulePriority=Speed  RndMeth=Simplest
      settings: InputPortMap=u0,u1,u2
  2-D Lookup Table19 : Lookup_n-D  NumberOfTableDimensions=3  LookupTableObject=''  BreakpointsForDimension1=db.aerody.VH  BreakpointsForDimension2=db.aerody.VALPHA  BreakpointsForDimension3=db.aerody.VDF  BreakpointsForDimension1FirstPoint=10  BreakpointsForDimension2FirstPoint=10  BreakpointsForDimension1Spacing=12  BreakpointsForDimension2Spacing=12  IndexSearchMethod=Linear search  BeginIndexSearchUsingPreviousIndexResult=on  Table=db.aerody.CLHDFRO  ExtrapMethod=Clip  DiagnosticForOutOfRangeInput=Warning  InternalRulePriority=Speed  RndMeth=Simplest
      settings: InputPortMap=u0,u1,u2
  2-D Lookup Table2 : Lookup_n-D  LookupTableObject=''  BreakpointsForDimension1=db.aerody.VDF  BreakpointsForDimension2=db.aerody.VALPHA  BreakpointsForDimension1FirstPoint=10  BreakpointsForDimension2FirstPoint=10  BreakpointsForDimension1Spacing=12  BreakpointsForDimension2Spacing=12  IndexSearchMethod=Linear search  BeginIndexSearchUsingPreviousIndexResult=on  Table=db.aerody.CLDFRI  ExtrapMethod=Clip  DiagnosticForOutOfRangeInput=Warning  InternalRulePriority=Speed  RndMeth=Simplest
      settings: InputPortMap=u0,u1
  2-D Lookup Table20 : Lookup_n-D  LookupTableObject=''  BreakpointsForDimension1=db.aerody.VTC  BreakpointsForDimension2=db.aerody.VALPHA  BreakpointsForDimension1FirstPoint=10  BreakpointsForDimension2FirstPoint=10  BreakpointsForDimension1Spacing=12  BreakpointsForDimension2Spacing=12  IndexSearchMethod=Linear search  BeginIndexSearchUsingPreviousIndexResult=on  Table=db.aerody.CLSS  ExtrapMethod=Clip  DiagnosticForOutOfRangeInput=Warning  InternalRulePriority=Speed  RndMeth=Simplest
      settings: InputPortMap=u0,u1
  2-D Lookup Table3 : Lookup_n-D  LookupTableObject=''  BreakpointsForDimension1=db.aerody.VDF  BreakpointsForDimension2=db.aerody.VALPHA  BreakpointsForDimension1FirstPoint=10  BreakpointsForDimension2FirstPoint=10  BreakpointsForDimension1Spacing=12  BreakpointsForDimension2Spacing=12  IndexSearchMethod=Linear search  BeginIndexSearchUsingPreviousIndexResult=on  Table=db.aerody.CLDFRO  ExtrapMethod=Clip  DiagnosticForOutOfRangeInput=Warning  InternalRulePriority=Speed  RndMeth=Simplest
      settings: InputPortMap=u0,u1
  2-D Lookup Table4 : Lookup_n-D  LookupTableObject=''  BreakpointsForDimension1=db.aerody.VDA  BreakpointsForDimension2=db.aerody.VALPHA  BreakpointsForDimension1FirstPoint=10  BreakpointsForDimension2FirstPoint=10  BreakpointsForDimension1Spacing=12  BreakpointsForDimension2Spacing=12  IndexSearchMethod=Linear search  BeginIndexSearchUsingPreviousIndexResult=on  Table=db.aerody.CLDAL  ExtrapMethod=Clip  DiagnosticForOutOfRangeInput=Warning  InternalRulePriority=Speed  RndMeth=Simplest
      settings: InputPortMap=u0,u1
  2-D Lookup Table5 : Lookup_n-D  LookupTableObject=''  BreakpointsForDimension1=db.aerody.VDA  BreakpointsForDimension2=db.aerody.VALPHA  BreakpointsForDimension1FirstPoint=10  BreakpointsForDimension2FirstPoint=10  BreakpointsForDimension1Spacing=12  BreakpointsForDimension2Spacing=12  IndexSearchMethod=Linear search  BeginIndexSearchUsingPreviousIndexResult=on  Table=db.aerody.CLDAR  ExtrapMethod=Clip  DiagnosticForOutOfRangeInput=Warning  InternalRulePriority=Speed  RndMeth=Simplest
      settings: InputPortMap=u0,u1
  2-D Lookup Table6 : Lookup_n-D  LookupTableObject=''  BreakpointsForDimension1=db.aerody.VDF  BreakpointsForDimension2=db.aerody.VALPHA  BreakpointsForDimension1FirstPoint=10  BreakpointsForDimension2FirstPoint=10  BreakpointsForDimension1Spacing=12  BreakpointsForDimension2Spacing=12  IndexSearchMethod=Linear search  BeginIndexSearchUsingPreviousIndexResult=on  Table=db.aerody.CLDFLO  ExtrapMethod=Clip  DiagnosticForOutOfRangeInput=Warning  InternalRulePriority=Speed  RndMeth=Simplest
      settings: InputPortMap=u0,u1
  2-D Lookup Table7 : Lookup_n-D  NumberOfTableDimensions=1  LookupTableObject=''  BreakpointsForDimension1=db.aerody.VALPHA  BreakpointsForDimension2=aerody.basic.cx.beta  BreakpointsForDimension1FirstPoint=10  BreakpointsForDimension2FirstPoint=10  BreakpointsForDimension1Spacing=12  BreakpointsForDimension2Spacing=12  IndexSearchMethod=Linear search  BeginIndexSearchUsingPreviousIndexResult=on  Table=db.aerody.CLB  ExtrapMethod=Clip  DiagnosticForOutOfRangeInput=Warning  InternalRulePriority=Speed  RndMeth=Simplest
  2-D Lookup Table8 : Lookup_n-D  LookupTableObject=''  BreakpointsForDimension1=db.aerody.VDE  BreakpointsForDimension2=db.aerody.VALPHA  BreakpointsForDimension1FirstPoint=10  BreakpointsForDimension2FirstPoint=10  BreakpointsForDimension1Spacing=12  BreakpointsForDimension2Spacing=12  IndexSearchMethod=Linear search  BeginIndexSearchUsingPreviousIndexResult=on  Table=db.aerody.CLDEL  ExtrapMethod=Clip  DiagnosticForOutOfRangeInput=Warning  InternalRulePriority=Speed  RndMeth=Simplest
      settings: InputPortMap=u0,u1
  2-D Lookup Table9 : Lookup_n-D  LookupTableObject=''  BreakpointsForDimension1=db.aerody.VDE  BreakpointsForDimension2=db.aerody.VALPHA  BreakpointsForDimension1FirstPoint=10  BreakpointsForDimension2FirstPoint=10  BreakpointsForDimension1Spacing=12  BreakpointsForDimension2Spacing=12  IndexSearchMethod=Linear search  BeginIndexSearchUsingPreviousIndexResult=on  Table=db.aerody.CLDEM  ExtrapMethod=Clip  DiagnosticForOutOfRangeInput=Warning  InternalRulePriority=Speed  RndMeth=Simplest
      settings: InputPortMap=u0,u1
  Angle Conversion1 : aerolibconvert2/Angle Conversion  IU=rad  OU=deg
  Angle Conversion2 : aerolibconvert2/Angle Conversion  IU=rad  OU=deg
  Gain : Gain
  Product : Product
  Saturation : Saturate  UpperLimit=5.8  LowerLimit=0
  Sum : Sum  Inputs=19
  CL : Outport
  wires:
  BusElementIn7/1 -> 2-D Lookup Table16/3, 2-D Lookup Table1/1
  BusElementIn1/1 -> 2-D Lookup Table17/3, 2-D Lookup Table6/1
  BusElementIn2/1 -> 2-D Lookup Table18/3, 2-D Lookup Table2/1
  BusElementIn3/1 -> 2-D Lookup Table19/3, 2-D Lookup Table3/1
  BusElementIn4/1 -> 2-D Lookup Table4/1
  BusElementIn5/1 -> 2-D Lookup Table5/1
  BusElementIn6/1 -> 2-D Lookup Table8/1
  BusElementIn8/1 -> 2-D Lookup Table9/1
  BusElementIn9/1 -> 2-D Lookup Table10/1
  BusElementIn10/1 -> 2-D Lookup Table13/1, 2-D Lookup Table12/1
  BusElementIn12/1 -> Angle Conversion2/1
  2-D Lookup Table/1 -> Product/1
  BusElementIn13/1 -> Saturation/1
  TC/1 -> 2-D Lookup Table20/1
  BusElementIn/1 -> Angle Conversion1/1
  2-D Lookup Table2/1 -> Sum/10  "CLDFRI"
  2-D Lookup Table4/1 -> Sum/12  "CLDAL"
  2-D Lookup Table3/1 -> Sum/11  "CLDFRO"
  2-D Lookup Table1/1 -> Sum/8  "CLDFLI"
  2-D Lookup Table6/1 -> Sum/9  "CLDFLO"
  2-D Lookup Table8/1 -> Sum/14  "CLDEL"
  2-D Lookup Table18/1 -> Sum/6  "CLHDFRI"
  2-D Lookup Table5/1 -> Sum/13  "CLDAR"
  2-D Lookup Table19/1 -> Sum/7  "CLHDFRO"
  2-D Lookup Table10/1 -> Sum/16  "CLDER"
  2-D Lookup Table16/1 -> Sum/4  "CLHDFLI"
  2-D Lookup Table9/1 -> Sum/15  "CLDEM"
  2-D Lookup Table17/1 -> Sum/5  "CLHDFLO"
  2-D Lookup Table12/1 -> Sum/17  "CLDR"
  2-D Lookup Table20/1 -> Sum/2  "CLSS"
  Product/1 -> Sum/18  "DCLBETA*BETA"
  2-D Lookup Table15/1 -> Sum/3  "CLH"
  2-D Lookup Table7/1 -> Sum/1  "CLB"
  2-D Lookup Table13/1 -> Sum/19  "CLDRBETA"
  Sum/1 -> Gain/1  "CL1"
  Gain/1 -> CL/1
  Saturation/1 -> 2-D Lookup Table19/1, 2-D Lookup Table18/1, 2-D Lookup Table17/1, 2-D Lookup Table16/1, 2-D Lookup Table15/1
  Angle Conversion1/1 -> 2-D Lookup Table12/2, 2-D Lookup Table13/2, 2-D Lookup Table/2, 2-D Lookup Table10/2, 2-D Lookup Table9/2, 2-D Lookup Table8/2, 2-D Lookup Table5/2, 2-D Lookup Table4/2, 2-D Lookup Table3/2, 2-D Lookup Table2/2, 2-D Lookup Table6/2, 2-D Lookup Table1/2, 2-D Lookup Table19/2, 2-D Lookup Table18/2, 2-D Lookup Table17/2, 2-D Lookup Table16/2, 2-D Lookup Table15/2, 2-D Lookup Table20/2, 2-D Lookup Table7/1
  Angle Conversion2/1 -> 2-D Lookup Table13/3, Product/2, 2-D Lookup Table/1
